simulink model "sldemo_tc"  (Simulink 6.0)
settings: Solver=ode3  SolverMode=SingleTasking  StartTime=0.0  StopTime=10.0  FixedStep=0.005  RelTol=1e-3
PreLoadFcn:
  | load sldemo_tc_data.mat
model workspace: external: M-Code (data not in the file)
values from neighbouring files (symbols this model uses):
  TypeS_bits_bp = single(TypeS_bits_bp)    [sldemo_create_tc_tabledata.m]    (also in sldemo_tc_data.mat = [0 50 100 150 200 250 300 350 400 450 500 550 ... (83 elemen)
  TypeS_tdegc_vs_bits = single(interp1(es,ts,e_vs_counts, 'linear','extrap'))    [sldemo_create_tc_tabledata.m]    (also in sldemo_tc_data.mat = [-50 -48.8466186523 -47.6932373047 -46.6318855286 -45.636474)
libraries: simulink x3, simulink_extras x1
settings Model: Creator=The MathWorks Inc.  LastModifiedBy=batserve  ExtModeAutoUpdateStatusClock=off  ProdHWDeviceType=32-bit xPC Target (AMD Athlon)
settings DataIOCC: SaveOutput=off  SaveTime=off
settings OptimizationCC: InlineParams=on
settings DebuggingCC: CheckExecutionContextPreStartOutputMsg=on  CheckExecutionContextRuntimeOutputMsg=on
settings HardwareCC: ProdIntDivRoundTo=Floor  ProdEndianess=LittleEndian  ProdHWDeviceType=32-bit xPC Target (AMD Athlon)
settings RTWCC: GenCodeOnly=on
settings GRTTargetCC: TargetFcnLib=iso_tfl_tmw.mat  GenFloatMathFcnCalls=ISO_C

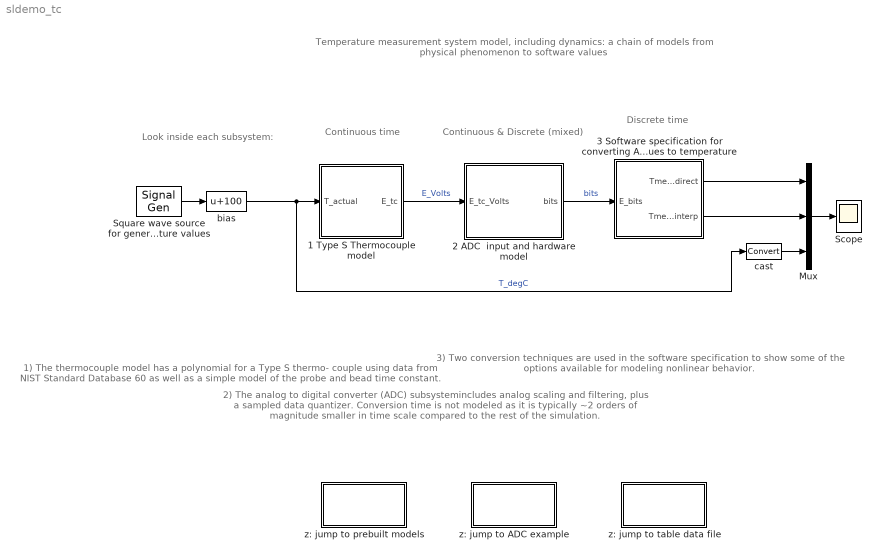
== system sldemo_tc ==
  note: Temperature measurement system model, including dynamics:
      | a chain of models from physical phenomenon to software values
  note: 1) The thermocouple model has
      | a polynomial for a Type S thermo-
      | couple using data from NIST
      | Standard Database 60 as well
      | as a simple model of the probe
      | and bead time constant.
  note: 2) The analog to digital converter
      | (ADC) subsystemincludes analog
      | scaling and filtering, plus a
      | sampled data quantizer.
      | Conversion time is not modeled
      | as it is typically ~2 orders of
      | magnitude smaller in time scale
      | compared to the rest of the
      | simulation.
  note: 3) Two conversion techniques
      | are used  in the software
      | specification to show some
      | of the options available for
      | modeling nonlinear behavior.
  note: Continuous
      | time
  note: Discrete
      | time
  note: Continuous &
      | Discrete (mixed)
  note: Look inside
      | each subsystem:
  1 Type S Thermocouple model : Subsystem  PropExecContextAcrossSSBoundary=on
  2 ADC  input and hardware model : Subsystem  PropExecContextAcrossSSBoundary=on
  3 Software specification for converting ADC values to temperature : Subsystem  PropExecContextAcrossSSBoundary=on
  Mux : Mux  Inputs=3
  Scope : Scope
      settings: TimeRange=10  YMin=-25  YMax=225
  Square wave source for generating temperature values : SignalGenerator  WaveForm=square  Amplitude=100
  bias : Bias  Bias=100
  cast : DataTypeConversion  OutDataTypeMode=single
  z: jump to ADC example : Subsystem  PropExecContextAcrossSSBoundary=on
      settings: OpenFcn=open_system('sldemo_adc_quantize','force')
      mask Type: ADC quantizer details
      mask Description: Jump to a model that exercises more details of the behavior of the Idealized ADC quantizer block that is part of the hardware model.
      mask Display: disp('ADC Quantizer\nDetails')
  z: jump to prebuilt models : Subsystem  PropExecContextAcrossSSBoundary=on
      settings: OpenFcn=open_system('sldemo_tc_blocks','force')
      mask Type: ADC quantizer details
      mask Description: Jump to a model that exercises more details of the behavior of the Idealized ADC quantizer block that is part of the hardware model.
      mask Display: disp('Additional\nThermocouple\nModels')
  z: jump to table data file : Subsystem  PropExecContextAcrossSSBoundary=on
      settings: OpenFcn=edit sldemo_create_tc_tabledata.m
      mask Type: ADC quantizer details
      mask Description: Jump to a model that exercises more details of the behavior of the Idealized ADC quantizer block that is part of the hardware model.
      mask Display: disp('Table Design\nDetails')
  wires:
  3 Software specification for converting ADC values to temperature/1(Tmeas_direct) -> Mux/1
  1 Type S Thermocouple model/1(E_tc) -> 2 ADC  input and hardware model/1(E_tc_Volts)  "E_Volts"
  2 ADC  input and hardware model/1(bits) -> 3 Software specification for converting ADC values to temperature/1(E_bits)  "bits"
  3 Software specification for converting ADC values to temperature/2(Tmeas_interp) -> Mux/2
  Mux/1 -> Scope/1
  bias/1 -> 1 Type S Thermocouple model/1(T_actual), cast/1  "T_degC"
  Square wave source for generating temperature values/1 -> bias/1
  cast/1 -> Mux/3

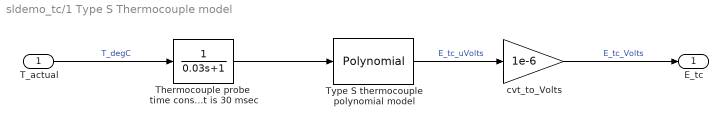
== system sldemo_tc/1 Type S Thermocouple model ==
  T_actual : Inport  Port=1  LatchInput=off
  Thermocouple probe  time constant is 30 msec : TransferFcn  Denominator=[0.03 1]
  Type S thermocouple polynomial model : simulink/Math Operations/Polynomial  Description=|  coefs=[ +2.71443176145e-021, -1.25068871393e-017, +2.55744251786e-014, -3.31465196389e-011, +3.22028823036e-008, -2.32477968689e-005, +1.25934289740e-002, +5.40313308631e+000, +0.00000000000e+000 ]
      | 0 deg C ice reference         
      |       microVolts = f(Temperature degC)   
      | (Segment 1) input range: -50 to 1063 degC
      settings: AttributesFormatString=%<Description>
  cvt_to_Volts : Gain  Gain=1e-6
  E_tc : Outport
  wires:
  Thermocouple probe  time constant is 30 msec/1 -> Type S thermocouple polynomial model/1
  T_actual/1 -> Thermocouple probe  time constant is 30 msec/1  "T_degC"
  Type S thermocouple polynomial model/1 -> cvt_to_Volts/1  "E_tc_uVolts"
  cvt_to_Volts/1 -> E_tc/1  "E_tc_Volts"

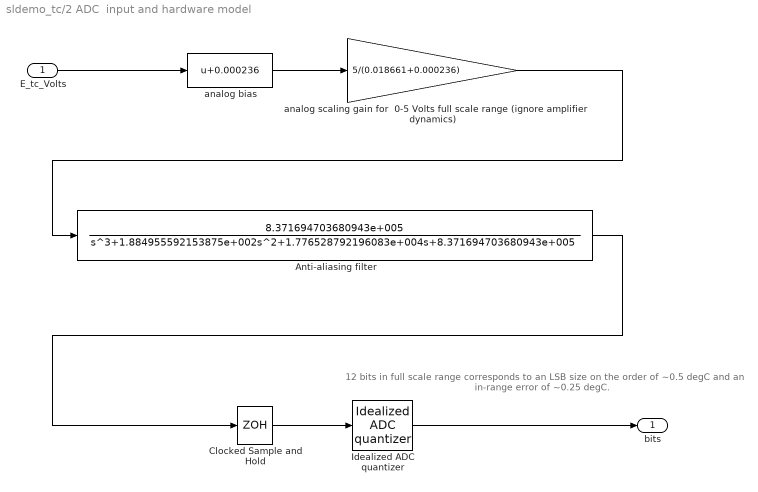
== system sldemo_tc/2 ADC  input and hardware model ==
  note: 12 bits in full scale range corresponds to
      | an LSB size on the order of ~0.5 degC and
      | an in-range error of ~0.25 degC.
  E_tc_Volts : Inport  Port=1  LatchInput=off
  Anti-aliasing filter : TransferFcn  Description=|  Numerator=8.371694703680943e+005  Denominator=[ 1, 1.884955592153875e+002, 1.776528792196083e+004, 8.371694703680943e+005 ]
      | Designed using Signal Processing Toolbox command:
      | >> [num,den] = butter(3,15*2*pi,'low','s')
      settings: AttributesFormatString=%<Description>
  Clocked Sample and Hold : ZeroOrderHold  SampleTime=0.020
      settings: AttributesFormatString=(%<SampleTime> sec)
  Idealized ADC quantizer : simulink_extras/Additional Discrete/Idealized ADC quantizer  NumberOfConverterBits=12  Vmin=0  Vmax=5  OutputDataType=uint16  OutputNegativeValues=off
  analog bias : Bias  Bias=0.000236
  analog scaling gain for  0-5 Volts full scale range (ignore amplifier dynamics) : Gain  Gain=5/(0.018661+0.000236)
  bits : Outport
  wires:
  analog scaling gain for  0-5 Volts full scale range (ignore amplifier dynamics)/1 -> Anti-aliasing filter/1
  E_tc_Volts/1 -> analog bias/1
  Clocked Sample and Hold/1 -> Idealized ADC quantizer/1
  Idealized ADC quantizer/1 -> bits/1
  analog bias/1 -> analog scaling gain for  0-5 Volts full scale range (ignore amplifier dynamics)/1
  Anti-aliasing filter/1 -> Clocked Sample and Hold/1

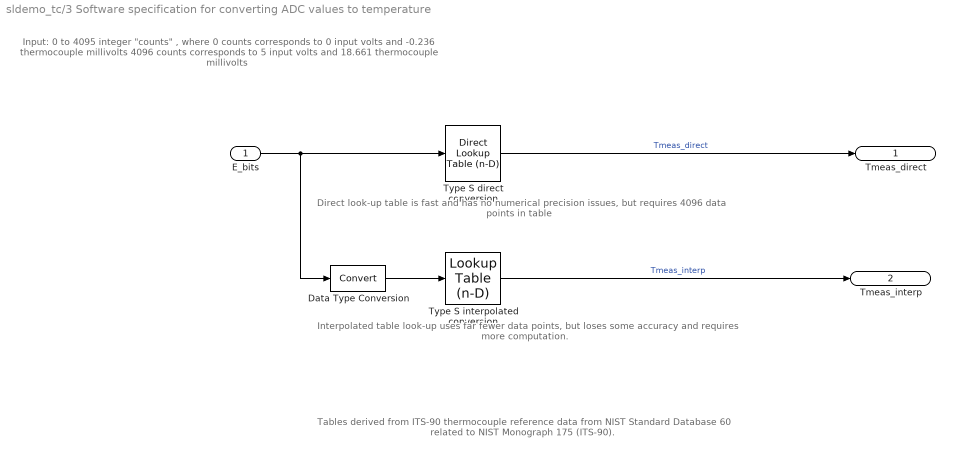
== system sldemo_tc/3 Software specification for converting ADC values to temperature ==
  note: Input: 0 to 4095 integer "counts" , where
      |             0        counts corresponds to 0 input volts and -0.236 thermocouple millivolts
      |             4096 counts corresponds to 5 input volts and 18.661 thermocouple millivolts
  note: Tables derived from ITS-90 thermocouple reference data
      | from NIST Standard Database 60 related to NIST Monograph 175 (ITS-90).
  note: Direct look-up table is fast and has no numerical precision issues,
      | but requires 4096 data points in table
  note: Interpolated table look-up uses far fewer data points,
      | but loses some accuracy and requires more computation.
  E_bits : Inport  Port=1  DataType=uint16  LatchInput=off
  Data Type Conversion : DataTypeConversion  OutDataTypeMode=single
  Type S direct conversion : simulink/Lookup Tables/Direct Lookup Table (n-D)  maskTabDims=1  explicitNumDims=1  outDims=Element  tabIsInput=off  mxTable=TypeS_tdegc_vs_bits  clipFlag=Warning
      settings: AttributesFormatString=(%<mxTable>)
  Type S interpolated conversion : simulink/Lookup Tables/Lookup Table (n-D)  numDimsPopupSelect=1  bp1=TypeS_bits_bp  bp2=[10,22,31]  bp3=[1:3]  bp4=[1:3]  bpcell={ [1:3], [1:3] }  explicitNumDims=2  searchMode=Linear Search  cacheBpFlag=on  vectorInputFlag=off  tableData=TypeS_tdegc_interp  interpMethod=Linear  extrapMethod=None - Clip  rangeErrorMode=Warning
      settings: AttributesFormatString=(%<tableData>)
  Tmeas_direct : Outport
  Tmeas_interp : Outport  Port=2
  wires:
  E_bits/1 -> Type S direct conversion/1, Data Type Conversion/1
  Type S direct conversion/1 -> Tmeas_direct/1  "Tmeas_direct"
  Data Type Conversion/1 -> Type S interpolated conversion/1
  Type S interpolated conversion/1 -> Tmeas_interp/1  "Tmeas_interp"

== system sldemo_tc/z: jump to ADC example ==
  note: This block intentionally has no contents.

== system sldemo_tc/z: jump to prebuilt models ==
  note: This block intentionally has no contents.

== system sldemo_tc/z: jump to table data file ==
  note: This block intentionally has no contents.
